simulink model "part3"  (R2015a)
settings: Solver=ode1  StartTime=0.0  StopTime=100  FixedStep=0.1  RelTol=1e-8
libraries: simulink x1
settings Model: Creator=vdrouinv  LastModifiedBy=vdrouinv

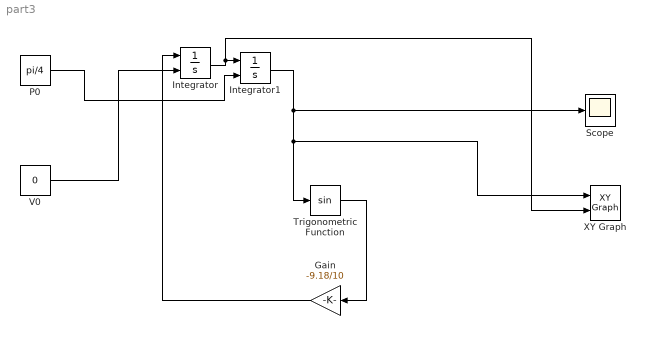
== system part3 ==
  Gain : Gain  Gain=-9.18/10
  Integrator : Integrator  InitialConditionSource=external
  Integrator1 : Integrator  InitialConditionSource=external
  P0 : Constant  Value=pi/4
  Scope : Scope
  Trigonometric Function : Trigonometry
  V0 : Constant  Value=0
  XY Graph : simulink/Sinks/XY Graph  xmin=-100  xmax=1  ymin=-5  ymax=5  st=-1
  wires:
  Trigonometric Function/1 -> Gain/1
  Integrator/1 -> XY Graph/2, Integrator1/1
  Integrator1/1 -> Scope/1, XY Graph/1, Trigonometric Function/1
  Gain/1 -> Integrator/1
  P0/1 -> Integrator1/2
  V0/1 -> Integrator/2
